simulink model "ecvt_model_lookup"  (R2023b)
settings: Solver=VariableStepAuto  StartTime=0.0  StopTime=10.0  RelTol=1e-3
libraries: fl_lib x4, sdl_lib x2, slpidlib x1, nesl_utility x1
settings Model: Creator=aarishadeel  LastModifiedBy=aarishadeel

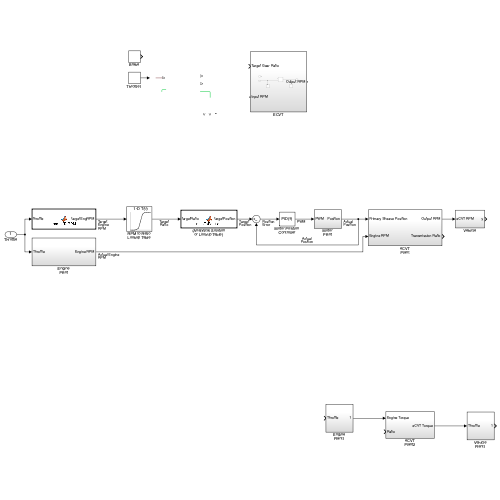
[thumbnail: Simulink's stored preview of the top-level diagram]
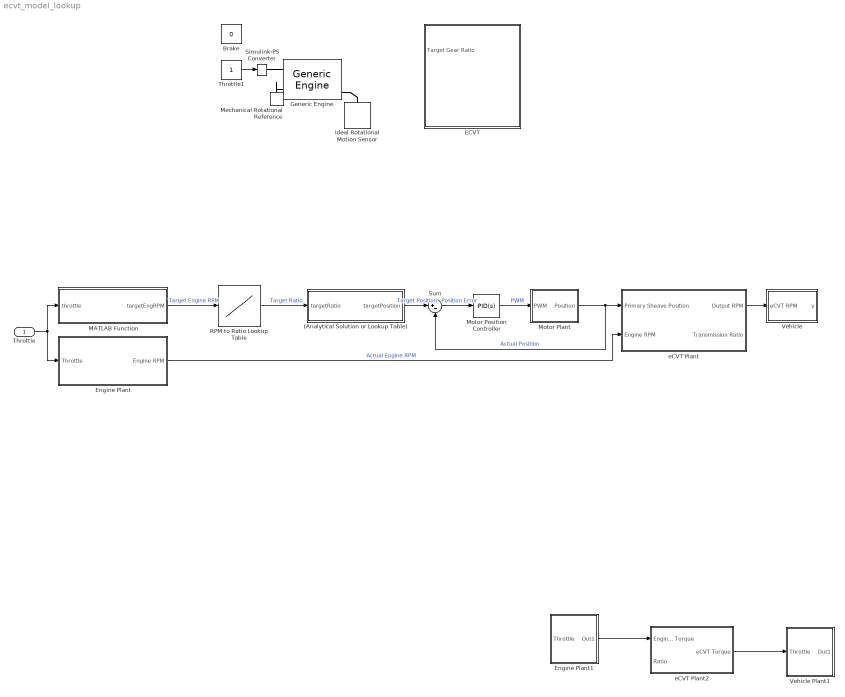
== system ecvt_model_lookup ==
  Throttle : Inport
  (Analytical Solution or Lookup Table) : MATLAB Function  TreatAsAtomicUnit=on
  Brake : Constant  Value=0
  ECVT : Subsystem
  Engine Plant : Subsystem
  Engine Plant1 : Subsystem
  Generic Engine : sdl_lib/Engines & Motors/Generic Engine  input_type=sdl.enum.GenericEngineInputType.NormalizedThrottle  model_parameterization=sdl.enum.engineParameterization.polynomial  engine_type=sdl.enum.engineType.SI  Trq_max=380 N*m  w_Trq_max=4300 rpm  P_max=230 kW  w_P_max=6858 rpm  w_max=7000 rpm  w_min=500 rpm  w_tab=[500, 1000, 2000, 3000, 4300, 5000, 6000, 7000] rpm  trq_tab=[250, 280, 330, 360, 380, 370, 350, 310] N*m  pwr_tab=[10, 30, 70, 110, 165, 190, 220, 230] kW  interp_method=simscape.enum.interpolation.linear  w_thr=100 rpm  model_inertia=sdl.enum.model_inertia.off  inertia=1 kg*m^2  initial_velocity=800 rpm  model_time_constant=sdl.enum.lagOffOn.off  time_constant=0.2 s  initial_normalized_throttle=0  fc_model=sdl.enum.fuel_consumption_model.FuelOff  fc_per_rev=25 mg/rev  fc_w_tab=[1000, 2000, 3000, 4000, 5000, 6000] rpm  fc_trq_tab=[0, 80, 160, 200, 240, 320, 360, 400] N*m  fc_tab=[.5, .9, 1.4, 1.6, 1.9, 2.7, 3.4, 4.4; 1, 1.7, 2.7, 3.1, 3.6, 5, 6, 7.4; 1.4, 2.7, 4, 4.8, 5.6, 7.5, 8.5, 10.5; 2, 3.6, 5.8, 6.7, 8, 10.4, 11.7, 13.3; 2.5, 4.8, 7.9, 9.4, 10.8, 14, 16.2, 18.6; 3.1, 6, 10.3, 11.9, 13.8, 18.4, 22, 26.5] g/s  bmep_tab=[0, 250, 500, 625, 750, 1000, 1150, 1250] kPa  bsfc_tab=[410, 380, 300, 280, 270, 290, 320, 380; 410, 370, 290, 270, 260, 270, 285, 320; 415, 380, 290, 275, 265, 270, 270, 300; 420, 390, 310, 290, 285, 280, 280, 285; 430, 410, 340, 320, 310, 300, 310, 320; 450, 430, 370, 340, 330, 330, 350, 380] g/(hr*kW)  fc_interp_method=simscape.enum.interpolation.linear  displaced_volume=400 cm^3  rev_per_cycle=2  idle_speed=false  idle_speed_reference=1000 rpm  tau_controller=1 s  idle_w_thr=1 rpm  redline=false  redline_speed=5000 rpm  tau_redline=1 s  redline_w_thr=1 rpm
      settings: InternalSimscapePortConfiguration="{\"Bottom\":[],\"Left\":[{\"id\":\"ThrNorm\",\"label\":\"Thr\",\"type\":\"input\"},{\"id\":\"B\",\"label\":\"B\",\"type\":\"foundation.mechanical.rotational.rotational\"}],\"Right\":[{\"id\":\"P\",\"label\":\"P\",\"type\":\"output\"},{\"id\":\"FC\",\"label\":\"FC\",\"type\":\"output\"},{\"id\":\"F\",\"label\":\"F\",\"type\":\"foundation.mechanical.rotational.rotational\"}],\"Top\":[]}"
  Ideal Rotational Motion Sensor : fl_lib/Mechanical/Mechanical Sensors/Ideal Rotational Motion Sensor  reference=foundation.enum.MeasurementReference.difference  acceleration_port=false  velocity_port=true  position_port=true  wrap_angle=false  offset=0 rad
  MATLAB Function : MATLAB Function  TreatAsAtomicUnit=on
  Mechanical Rotational Reference : fl_lib/Mechanical/Rotational Elements/Mechanical Rotational Reference
  Motor Plant : Subsystem
  Motor Position Controller : slpidlib/PID Controller  Controller=PID  Form=Parallel  TimeDomain=Continuous-time  UseExternalTs=off  SampleTime=-1  IntegratorMethod=Forward Euler  FilterMethod=Forward Euler  ControllerParametersSource=internal  P=1  I=1  UseKiTs=off  D=0  N=100  UseFilter=on  TunerSelectOption=Transfer Function Based (PID Tuner App)  InitialConditionSource=internal  InitialConditionForIntegrator=0  InitialConditionForFilter=0  DifferentiatorICPrevScaledInput=0  ExternalReset=none  TrackingMode=off  Kt=1  LimitOutput=off  SatLimitsSource=internal  UpperSaturationLimit=inf  LowerSaturationLimit=-inf  LinearizeAsGain=on  AntiWindupMode=none  Kb=1  LimitIntegrator=off  UpperIntegratorSaturationLimit=inf  LowerIntegratorSaturationLimit=-inf  POutMin=[]  POutMax=[]  IOutMin=[]  IOutMax=[]  DOutMin=[]  DOutMax=[]  NOutMin=[]  NOutMax=[]  SumOutMin=[]  SumOutMax=[]  SaturationOutMin=[]  SaturationOutMax=[]  PParamMin=[]  PParamMax=[]  IParamMin=[]  IParamMax=[]  DParamMin=[]  DParamMax=[]  NParamMin=[]  NParamMax=[]  KbParamMin=[]  KbParamMax=[]  KtParamMin=[]  KtParamMax=[]  KbOutMin=[]  KbOutMax=[]  KtOutMin=[]  KtOutMax=[]  IntegratorOutMin=[]  IntegratorOutMax=[]  FilterOutMin=[]  FilterOutMax=[]  SumI1OutMin=[]  SumI1OutMax=[]  SumI2OutMin=[]  SumI2OutMax=[]  SumI3OutMin=[]  SumI3OutMax=[]  SumI4OutMin=[]  SumI4OutMax=[]  SumDOutMin=[]  SumDOutMax=[]  DifferentiatorOutMin=[]  DifferentiatorOutMax=[]  FilterDiffOutCoefMin=[]  FilterDiffOutCoefMax=[]  ReciprocalOutMin=[]  ReciprocalOutMax=[]  SumDenOutMin=[]  SumDenOutMax=[]  SumNumOutMin=[]  SumNumOutMax=[]  DivideOutMin=[]  DivideOutMax=[]  UdiffTsProdOutMin=[]  UdiffTsProdOutMax=[]  NTsProdOutMin=[]  NTsProdOutMax=[]  UintegralTsProdOutMin=[]  UintegralTsProdOutMax=[]  UngainTsProdOutMin=[]  UngainTsProdOutMax=[]  ClampingZeroOutDataTypeStr=Inherit: Inherit via back propagation  ClampingZeroOutMin=[]  ClampingZeroOutMax=[]  FilterDenConstantOutDataTypeStr=Inherit: Inherit via back propagation  FilterDenConstantOutMin=[]  FilterDenConstantOutMax=[]  PCopyOutDataTypeStr=Inherit: Inherit via back propagation  PCopyOutMin=[]  PCopyOutMax=[]  NCopyOutDataTypeStr=Inherit: Inherit via back propagation  NCopyOutMin=[]  NCopyOutMax=[]  IntegratorContinuousStateAttributes=''  IntegratorStateMustResolveToSignalObject=off  IntegratorRTWStateStorageClass=Auto  FilterContinuousStateAttributes=''  FilterStateMustResolveToSignalObject=off  FilterRTWStateStorageClass=Auto  ParallelPVariant=InternalParameters  IdealPVariant=Disabled  IVariant=InternalParameters  DVariant=InternalParameters  IntegratorVariant=Continuous  SatVariant=Disabled  AWVariant=Passthrough  PCopyVariant=Disabled  TRVariant=Disabled  FdbkBlocksVariant=Forward  IdealPFdbkVariant=Disabled  SatFdbkVariant=Disabled  DerivativeFilterVariant=ContFilter  NVariant=InternalParameters  NCopyVariant=Disabled  FilterICVariant=InternalICsFilter  IntegratorICVariant=InternalICs  ExternalResetVariant=Disabled  TRSumVariant=Passthrough  SumFdbkVariant=Disabled  SumVariant=Sum_PID  TsampFilterVariant=InternalTs  TsampNgainVariant=Passthrough  TsampIntegralVariant=Disabled_SignalSpec  ExternalSaturationOutDataTypeStr=Inherit: Same as second input
  RPM to Ratio Lookup Table : Lookup_n-D  NumberOfTableDimensions=1  BreakpointsForDimension1=[-5:5]  Table=tanh([-5:5])  InternalRulePriority=Speed  RndMeth=Simplest
  Simulink-PS Converter : nesl_utility/Simulink-PS Converter  PhysicalDomain=network_engine_domain  SubClassName=ps_input  LeftPortType=input  RightPortType=output  PseudoPeriodic=off  Frequencies=[]  NoiseDistribution=none  NoiseParameters=[]  Unit=1  AffineConversion=off  FilteringAndDerivatives=provide  SimscapeFilterOrder=1  InputFilterTimeConstant=0.001  UdotUserProvided=0
  Sum : Sum  Inputs=|+-
  Throttle1 : Constant
  Vehicle : Subsystem
  Vehicle Plant1 : Subsystem
  eCVT Plant : Subsystem
  eCVT Plant2 : Subsystem
  wires:
  Throttle1/1 -> Simulink-PS Converter/1
  Throttle/1 -> MATLAB Function/1(throttle), Engine Plant/1(Throttle)
  Sum/1 -> Motor Position Controller/1  "Position Error"
  Motor Position Controller/1 -> Motor Plant/1(PWM)  "PWM"
  Motor Plant/1(Position) -> eCVT Plant/1(Primary Sheave Position), Sum/2  "Actual Position"
  (Analytical Solution or Lookup Table)/1(targetPosition) -> Sum/1  "Target Position"
  MATLAB Function/1(targetEngRPM) -> RPM to Ratio Lookup Table/1  "Target Engine RPM"
  eCVT Plant/1(Output RPM) -> Vehicle/1(eCVT RPM)
  Engine Plant1/1(Out1) -> eCVT Plant2/1(Engine Torque)
  eCVT Plant2/1(eCVT Torque) -> Vehicle Plant1/1(Throttle)
  Engine Plant/1(Engine RPM) -> eCVT Plant/2(Engine RPM)  "Actual Engine RPM"
  RPM to Ratio Lookup Table/1 -> (Analytical Solution or Lookup Table)/1(targetRatio)  "Target Ratio"
  connections:
  Generic Engine/LConn1 -- Simulink-PS Converter/RConn1
  Mechanical Rotational Reference/LConn1 -- Generic Engine/LConn2
  Generic Engine/RConn3 -- Ideal Rotational Motion Sensor/LConn1

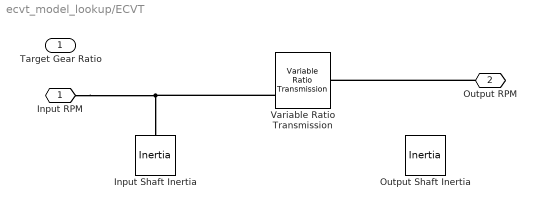
== system ecvt_model_lookup/ECVT ==
  Target Gear Ratio : Inport
  Input Shaft Inertia : fl_lib/Mechanical/Rotational Elements/Inertia  inertia=0.01 kg*m^2  num_ports=foundation.enum.numPorts2.one  w_specify=off  w_priority=High  w=0 rad/s  w_nominal_specify=off  w_nominal_unit=rad/s  w_nominal_value=1  t_specify=off  t_priority=None  t=0 N*m  t_nominal_specify=off  t_nominal_unit=N*m  t_nominal_value=1
  Output Shaft Inertia : fl_lib/Mechanical/Rotational Elements/Inertia  inertia=0.01 kg*m^2  num_ports=foundation.enum.numPorts2.one  w_specify=off  w_priority=High  w=0 rad/s  w_nominal_specify=off  w_nominal_unit=rad/s  w_nominal_value=1  t_specify=off  t_priority=None  t=0 N*m  t_nominal_specify=off  t_nominal_unit=N*m  t_nominal_value=1
  Variable Ratio Transmission : sdl_lib/Couplings & Drives/Variable Ratio Transmission  rotation_direction=sdl.enum.shaftOutputDirection.same  kp=3e5 N*m/rad  kv=0.05 N*m*s/rad  initial_torque=0 N*m  losses_model=sdl.enum.lossesOffOn.off  efficiency=0.8  w_thr=0.01 rad/s  mu_visc=[0, 0] N*m*s/rad  R_specify=off  R_priority=None  R=1  R_nominal_specify=off  R_nominal_unit=1  R_nominal_value=1
      settings: InternalSimscapePortConfiguration="{\"Bottom\":[],\"Left\":[{\"id\":\"ratio\",\"label\":\"r\",\"type\":\"input\"},{\"id\":\"B\",\"label\":\"B\",\"type\":\"foundation.mechanical.rotational.rotational\"}],\"Right\":[{\"id\":\"F\",\"label\":\"F\",\"type\":\"foundation.mechanical.rotational.rotational\"}],\"Top\":[]}"
  Input RPM : PMIOPort  Side=Left
  Output RPM : PMIOPort  Port=2  Side=Right
  connections:
  Input RPM/RConn1 -- Input Shaft Inertia/LConn1 -- Variable Ratio Transmission/LConn2
  Output RPM/RConn1 -- Variable Ratio Transmission/RConn1

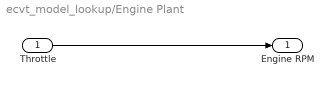
== system ecvt_model_lookup/Engine Plant ==
  Throttle : Inport
  Engine RPM : Outport
  wires:
  Throttle/1 -> Engine RPM/1

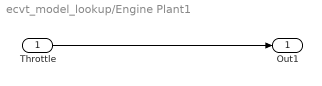
== system ecvt_model_lookup/Engine Plant1 ==
  Throttle : Inport
  Out1 : Outport
  wires:
  Throttle/1 -> Out1/1

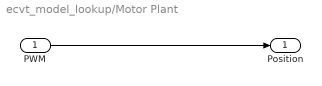
== system ecvt_model_lookup/Motor Plant ==
  PWM : Inport
  Position : Outport
  wires:
  PWM/1 -> Position/1

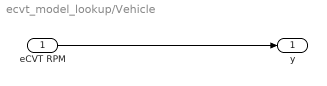
== system ecvt_model_lookup/Vehicle ==
  eCVT RPM : Inport
  y : Outport
  wires:
  eCVT RPM/1 -> y/1

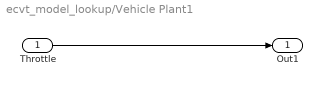
== system ecvt_model_lookup/Vehicle Plant1 ==
  Throttle : Inport
  Out1 : Outport
  wires:
  Throttle/1 -> Out1/1

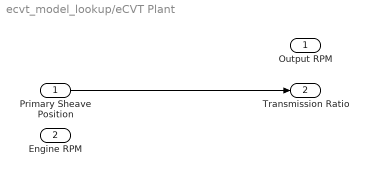
== system ecvt_model_lookup/eCVT Plant ==
  Primary Sheave Position : Inport
  Engine RPM : Inport  Port=2
  Output RPM : Outport
  Transmission Ratio : Outport  Port=2
  wires:
  Primary Sheave Position/1 -> Transmission Ratio/1

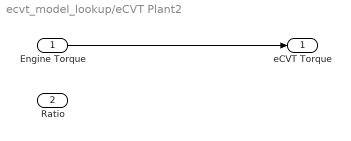
== system ecvt_model_lookup/eCVT Plant2 ==
  Engine Torque : Inport
  Ratio : Inport  Port=2
  eCVT Torque : Outport
  wires:
  Engine Torque/1 -> eCVT Torque/1

== matlab function ecvt_model_lookup/MATLAB Function ==
  data: throttle input; targetEngRPM output
function targetEngRPM = throttleToRPM(throttle)
%#codegen

targetEngineRPM = throttle;

== matlab function ecvt_model_lookup/(Analytical Solution or Lookup Table) ==
  data: targetRatio input; targetPosition output
function targetPosition = ratioToPosition(targetRatio)
%#codegen

y = u;
